simulink model "Cellmodel"  (Simulink 6.6)
settings: Solver=ode4  StartTime=0.0  StopTime=0.0001  FixedStep=0.000000001  RelTol=1e-3
(part 1 of 2)
settings Model: Creator=Thang M. Hoang  LastModifiedBy=Thang M. Hoang

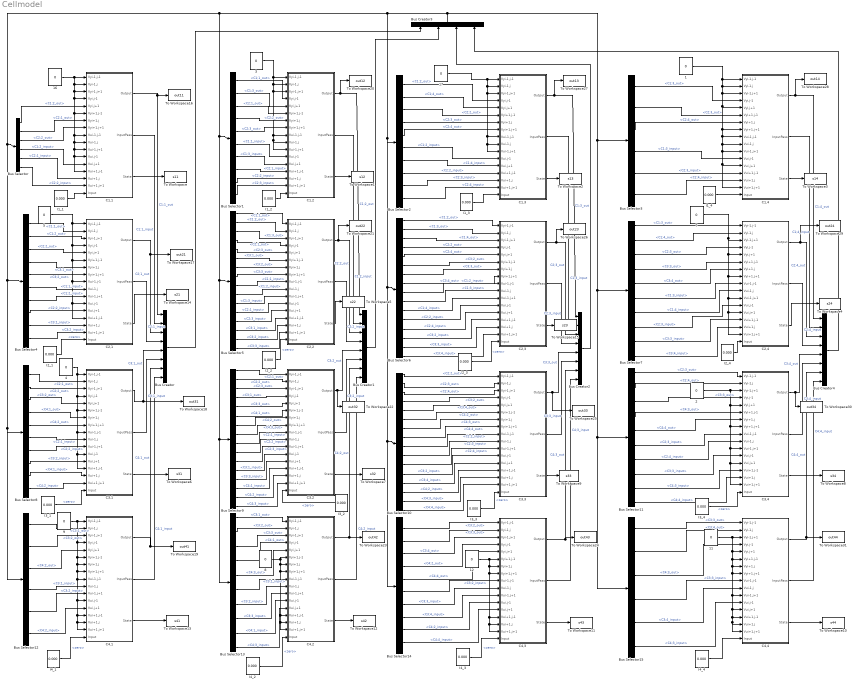
== system Cellmodel ==
  {1..5,7..9,11..12,16..17} (12 alike) : Constant  Value=0
  Bus Creator{,1..2,4} (4 alike) : BusCreator  Inputs=8
  Bus Creator3 : BusCreator  Orientation=up
  Bus Selector : BusSelector  OutputSignals=signal2.C1;2_out,signal1.C2;1_out,signal2.C2;2_out,signal2.C1;2_input,signal1.C2;1_input,signal2.C2;2_input
  Bus Selector1 : BusSelector  OutputSignals=signal1.C1;1_out,signal3.C1;3_out,signal1.C2;1_out,signal2.C2;2_out,signal3.C2;3_out,signal1.C1;1_input,signal3.C1;3_input,signal1.C2;1_input,signal2.C2;2_input,signal3.C2;3_input
  Bus Selector10 : BusSelector  OutputSignals=signal2.C2;2_out,signal3.C2;3_out,signal4.C2;4_out,signal2.C3;2_out,signal4.C3;4_out,signal2.C4;2_out,signal3.C4;3_out,signal4.C4;4_out,signal2.C2;2_input,signal3.C2;3_input,signal4.C2;4_input,signal2.C3;2_input,signal4.C3;4_input,signal2.C4;2_input,signal3.C4;3_input,signal4.C4;4_input
  Bus Selector11 : BusSelector  OutputSignals=signal3.C2;3_out,signal4.C2;4_out,signal3.C3;3_out,signal3.C4;3_out,signal4.C4;4_out,signal3.C2;3_input,signal4.C2;4_input,signal3.C3;3_input,signal3.C4;3_input,signal4.C4;4_input
  Bus Selector12 : BusSelector  OutputSignals=signal1.C3;1_out,signal2.C3;2_out,signal2.C4;2_out,signal1.C3;1_input,signal2.C3;2_input,signal2.C4;2_input
  Bus Selector13 : BusSelector  OutputSignals=signal1.C3;1_out,signal2.C3;2_out,signal3.C3;3_out,signal1.C4;1_out,signal3.C4;3_out,signal1.C3;1_input,signal2.C3;2_input,signal3.C3;3_input,signal1.C4;1_input,signal3.C4;3_input
  Bus Selector14 : BusSelector  OutputSignals=signal2.C3;2_out,signal3.C3;3_out,signal4.C3;4_out,signal2.C4;2_out,signal4.C4;4_out,signal2.C3;2_input,signal3.C3;3_input,signal4.C3;4_input,signal2.C4;2_input,signal4.C4;4_input
  Bus Selector15 : BusSelector  OutputSignals=signal3.C3;3_out,signal4.C3;4_out,signal3.C4;3_out,signal3.C3;3_input,signal4.C3;4_input,signal3.C4;3_input
  Bus Selector2 : BusSelector  OutputSignals=signal2.C1;2_out,signal4.C1;4_out,signal2.C2;2_out,signal3.C2;3_out,signal4.C2;4_out,signal2.C1;2_input,signal4.C1;4_input,signal2.C2;2_input,signal3.C2;3_input,signal4.C2;4_input
  Bus Selector3 : BusSelector  OutputSignals=signal3.C1;3_out,signal3.C2;3_out,signal4.C2;4_out,signal3.C1;3_input,signal3.C2;3_input,signal4.C2;4_input
  Bus Selector4 : BusSelector  OutputSignals=signal1.C1;1_out,signal2.C1;2_out,signal2.C2;2_out,signal1.C3;1_out,signal2.C3;2_out,signal1.C1;1_input,signal2.C1;2_input,signal2.C2;2_input,signal1.C3;1_input,signal2.C3;2_input
  Bus Selector5 : BusSelector  OutputSignals=signal1.C1;1_out,signal2.C1;2_out,signal3.C1;3_out,signal1.C2;1_out,signal3.C2;3_out,signal1.C3;1_out,signal2.C3;2_out,signal3.C3;3_out,signal1.C1;1_input,signal2.C1;2_input,signal3.C1;3_input,signal1.C2;1_input,signal3.C2;3_input,signal1.C3;1_input,signal2.C3;2_input,signal3.C3;3_input
  Bus Selector6 : BusSelector  OutputSignals=signal2.C1;2_out,signal3.C1;3_out,signal4.C1;4_out,signal2.C2;2_out,signal4.C2;4_out,signal2.C3;2_out,signal3.C3;3_out,signal4.C3;4_out,signal2.C1;2_input,signal3.C1;3_input,signal4.C1;4_input,signal2.C2;2_input,signal4.C2;4_input,signal2.C3;2_input,signal3.C3;3_input,signal4.C3;4_input
  Bus Selector7 : BusSelector  OutputSignals=signal3.C1;3_out,signal4.C1;4_out,signal3.C2;3_out,signal3.C3;3_out,signal4.C3;4_out,signal3.C1;3_input,signal4.C1;4_input,signal3.C2;3_input,signal3.C3;3_input,signal4.C3;4_input
  Bus Selector8 : BusSelector  OutputSignals=signal1.C2;1_out,signal2.C2;2_out,signal2.C3;2_out,signal1.C4;1_out,signal2.C4;2_out,signal1.C2;1_input,signal2.C2;2_input,signal2.C3;2_input,signal1.C4;1_input,signal2.C4;2_input
  Bus Selector9 : BusSelector  OutputSignals=signal1.C2;1_out,signal2.C2;2_out,signal3.C2;3_out,signal1.C3;1_out,signal3.C3;3_out,signal1.C4;1_out,signal2.C4;2_out,signal3.C4;3_out,signal1.C2;1_input,signal2.C2;2_input,signal3.C2;3_input,signal1.C3;1_input,signal3.C3;3_input,signal1.C4;1_input,signal2.C4;2_input,signal3.C4;3_input
  C1,1 : Subsystem
  C1,2 : Subsystem
  C1,3 : Subsystem
  C1,4 : Subsystem
  C2,1 : Subsystem
  C2,2 : Subsystem
  C2,3 : Subsystem
  C2,4 : Subsystem
  C3,1 : Subsystem
  C3,2 : Subsystem
  C3,3 : Subsystem
  C3,4 : Subsystem
  C4,1 : Subsystem
  C4,2 : Subsystem
  C4,3 : Subsystem
  C4,4 : Subsystem
  I1_{1..4} (4 alike) : Constant  Value=0.000
  I2_{1..4} (4 alike) : Constant  Value=0.000
  I3_1 : Constant  Value=0.000
  I3_2 : Constant  Orientation=left  Value=0.000
  I3_3 : Constant  Value=0.000
  I3_4 : Constant  Value=0.000
  I4_{1..4} (4 alike) : Constant  Value=0.000
  To Workspace : ToWorkspace  VariableName=s11  SampleTime=-1  SaveFormat=Array
  To Workspace1 : ToWorkspace  VariableName=s12  SampleTime=-1  SaveFormat=Array
  To Workspace10 : ToWorkspace  VariableName=s44  SampleTime=-1  SaveFormat=Array
  To Workspace11 : ToWorkspace  VariableName=s43  SampleTime=-1  SaveFormat=Array
  To Workspace12 : ToWorkspace  VariableName=s42  SampleTime=-1  SaveFormat=Array
  To Workspace13 : ToWorkspace  VariableName=s41  SampleTime=-1  SaveFormat=Array
  To Workspace14 : ToWorkspace  VariableName=s21  SampleTime=-1  SaveFormat=Array
  To Workspace15 : ToWorkspace  VariableName=s23  SampleTime=-1  SaveFormat=Array
  To Workspace16 : ToWorkspace  VariableName=out11  SampleTime=-1  SaveFormat=Array
  To Workspace17 : ToWorkspace  VariableName=out21  SampleTime=-1  SaveFormat=Array
  To Workspace18 : ToWorkspace  VariableName=out31  SampleTime=-1  SaveFormat=Array
  To Workspace19 : ToWorkspace  VariableName=out41  SampleTime=-1  SaveFormat=Array
  To Workspace2 : ToWorkspace  VariableName=s13  SampleTime=-1  SaveFormat=Array
  To Workspace20 : ToWorkspace  VariableName=out12  SampleTime=-1  SaveFormat=Array
  To Workspace21 : ToWorkspace  VariableName=out22  SampleTime=-1  SaveFormat=Array
  To Workspace22 : ToWorkspace  VariableName=out32  SampleTime=-1  SaveFormat=Array
  To Workspace23 : ToWorkspace  VariableName=out42  SampleTime=-1  SaveFormat=Array
  To Workspace24 : ToWorkspace  VariableName=out43  SampleTime=-1  SaveFormat=Array
  To Workspace25 : ToWorkspace  VariableName=out33  SampleTime=-1  SaveFormat=Array
  To Workspace26 : ToWorkspace  VariableName=out23  SampleTime=-1  SaveFormat=Array
  To Workspace27 : ToWorkspace  VariableName=out13  SampleTime=-1  SaveFormat=Array
  To Workspace28 : ToWorkspace  VariableName=out14  SampleTime=-1  SaveFormat=Array
  To Workspace29 : ToWorkspace  VariableName=out24  SampleTime=-1  SaveFormat=Array
  To Workspace3 : ToWorkspace  VariableName=s14  SampleTime=-1  SaveFormat=Array
  To Workspace30 : ToWorkspace  VariableName=out34  SampleTime=-1  SaveFormat=Array
  To Workspace31 : ToWorkspace  VariableName=out44  SampleTime=-1  SaveFormat=Array
  To Workspace4 : ToWorkspace  VariableName=s24  SampleTime=-1  SaveFormat=Array
  To Workspace5 : ToWorkspace  VariableName=s22  SampleTime=-1  SaveFormat=Array
  To Workspace6 : ToWorkspace  VariableName=s31  SampleTime=-1  SaveFormat=Array
  To Workspace7 : ToWorkspace  VariableName=s32  SampleTime=-1  SaveFormat=Array
  To Workspace8 : ToWorkspace  VariableName=s34  SampleTime=-1  SaveFormat=Array
  To Workspace9 : ToWorkspace  VariableName=s33  SampleTime=-1  SaveFormat=Array
  wires:
  C1,1/1(Output) -> Bus Creator/1, To Workspace16/1  "C1;1_out"
  C1,1/2(InputPass) -> Bus Creator/2  "C1;1_input"
  C2,1/1(Output) -> Bus Creator/3, To Workspace17/1  "C2;1_out"
  C2,1/2(InputPass) -> Bus Creator/4  "C2;1_input"
  C3,1/1(Output) -> Bus Creator/5, To Workspace18/1  "C3;1_out"
  C3,1/2(InputPass) -> Bus Creator/6  "C3;1_input"
  C4,1/1(Output) -> Bus Creator/7, To Workspace19/1  "C4;1_out"
  C4,1/2(InputPass) -> Bus Creator/8  "C4;1_input"
  C1,2/1(Output) -> Bus Creator1/1, To Workspace20/1  "C1;2_out"
  C1,2/2(InputPass) -> Bus Creator1/2  "C1;2_input"
  C2,2/1(Output) -> Bus Creator1/3, To Workspace21/1  "C2;2_out"
  C2,2/2(InputPass) -> Bus Creator1/4  "C2;2_input"
  C3,2/1(Output) -> Bus Creator1/5, To Workspace22/1  "C3;2_out"
  C3,2/2(InputPass) -> Bus Creator1/6  "C3;2_input"
  C4,2/1(Output) -> Bus Creator1/7, To Workspace23/1  "C4;2_out"
  C4,2/2(InputPass) -> Bus Creator1/8  "C4;2_input"
  C1,3/1(Output) -> Bus Creator2/1, To Workspace27/1  "C1;3_out"
  C1,3/2(InputPass) -> Bus Creator2/2  "C1;3_input"
  C2,3/1(Output) -> Bus Creator2/3, To Workspace26/1  "C2;3_out"
  C2,3/2(InputPass) -> Bus Creator2/4  "C2;3_input"
  C3,3/1(Output) -> Bus Creator2/5, To Workspace25/1  "C3;3_out"
  C3,3/2(InputPass) -> Bus Creator2/6  "C3;3_input"
  C4,3/1(Output) -> Bus Creator2/7, To Workspace24/1  "C4;3_out"
  C4,3/2(InputPass) -> Bus Creator2/8  "C4;3_input"
  C1,4/1(Output) -> Bus Creator4/1, To Workspace28/1  "C1;4_out"
  C1,4/2(InputPass) -> Bus Creator4/2  "C1;4_input"
  C2,4/1(Output) -> Bus Creator4/3, To Workspace29/1  "C2;4_out"
  C2,4/2(InputPass) -> Bus Creator4/4  "C2;4_input"
  C3,4/1(Output) -> Bus Creator4/5, To Workspace30/1  "C3;4_out"
  C3,4/2(InputPass) -> Bus Creator4/6  "C3;4_input"
  C4,4/1(Output) -> Bus Creator4/7, To Workspace31/1  "C4;4_out"
  C4,4/2(InputPass) -> Bus Creator4/8  "C4;4_input"
  Bus Creator/1 -> Bus Creator3/1
  Bus Creator1/1 -> Bus Creator3/2
  Bus Creator2/1 -> Bus Creator3/3
  Bus Creator4/1 -> Bus Creator3/4
  Bus Creator3/1 -> Bus Selector/1, Bus Selector4/1, Bus Selector8/1, Bus Selector12/1, Bus Selector1/1, Bus Selector5/1, Bus Selector9/1, Bus Selector13/1, Bus Selector2/1, Bus Selector6/1, Bus Selector10/1, Bus Selector14/1, Bus Selector3/1, Bus Selector7/1, Bus Selector11/1, Bus Selector15/1
  Bus Selector/2 -> C1,1/7(Vyi+1,j)  "<C2;1_out>"
  Bus Selector/5 -> C1,1/15(Vui+1,j)  "<C2;1_input>"
  Bus Selector/1 -> C1,1/5(Vyi,j+1)  "<C1;2_out>"
  Bus Selector/4 -> C1,1/13(Vui,j+1)  "<C1;2_input>"
  Bus Selector/3 -> C1,1/8(Vyi+1,j+1)  "<C2;2_out>"
  Bus Selector/6 -> C1,1/16(Vui+1,j+1)  "<C2;2_input>"
  Bus Selector1/1 -> C1,2/4(Vyi,j-1)  "<C1;1_out>"
  Bus Selector1/6 -> C1,2/12(Vui,j-1)  "<C1;1_input>"
  Bus Selector1/3 -> C1,2/6(Vyi+1,j-1)  "<C2;1_out>"
  Bus Selector1/8 -> C1,2/14(Vui+1,j-1)  "<C2;1_input>"
  Bus Selector1/4 -> C1,2/7(Vyi+1,j)  "<C2;2_out>"
  Bus Selector1/9 -> C1,2/15(Vui+1,j)  "<C2;2_input>"
  Bus Selector1/2 -> C1,2/5(Vyi,j+1)  "<C1;3_out>"
  Bus Selector1/7 -> C1,2/13(Vui,j+1)  "<C1;3_input>"
  Bus Selector1/5 -> C1,2/8(Vyi+1,j+1)  "<C2;3_out>"
  Bus Selector1/10 -> C1,2/16(Vui+1,j+1)  "<C2;3_input>"
  Bus Selector2/1 -> C1,3/4(Vyi,j-1)  "<C1;2_out>"
  Bus Selector2/3 -> C1,3/6(Vyi+1,j-1)  "<C2;2_out>"
  Bus Selector2/4 -> C1,3/7(Vyi+1,j)  "<C2;3_out>"
  Bus Selector2/2 -> C1,3/5(Vyi,j+1)  "<C1;4_out>"
  Bus Selector2/5 -> C1,3/8(Vyi+1,j+1)  "<C2;4_out>"
  Bus Selector2/6 -> C1,3/12(Vui,j-1)  "<C1;2_input>"
  Bus Selector2/8 -> C1,3/14(Vui+1,j-1)  "<C2;2_input>"
  Bus Selector2/9 -> C1,3/15(Vui+1,j)  "<C2;3_input>"
  Bus Selector2/7 -> C1,3/13(Vui,j+1)  "<C1;4_input>"
  Bus Selector2/10 -> C1,3/16(Vui+1,j+1)  "<C2;4_input>"
  Bus Selector3/1 -> C1,4/4(Vyi,j-1)  "<C1;3_out>"
  Bus Selector3/2 -> C1,4/6(Vyi+1,j-1)  "<C2;3_out>"
  Bus Selector3/3 -> C1,4/7(Vyi+1,j)  "<C2;4_out>"
  Bus Selector3/4 -> C1,4/12(Vui,j-1)  "<C1;3_input>"
  Bus Selector3/5 -> C1,4/14(Vui+1,j-1)  "<C2;3_input>"
  Bus Selector3/6 -> C1,4/15(Vui+1,j)  "<C2;4_input>"
  Bus Selector4/1 -> C2,1/2(Vyi-1,j)  "<C1;1_out>"
  Bus Selector4/4 -> C2,1/7(Vyi+1,j)  "<C3;1_out>"
  Bus Selector4/2 -> C2,1/3(Vyi-1,j+1)  "<C1;2_out>"
  Bus Selector4/3 -> C2,1/5(Vyi,j+1)  "<C2;2_out>"
  Bus Selector4/5 -> C2,1/8(Vyi+1,j+1)  "<C3;2_out>"
  Bus Selector4/6 -> C2,1/10(Vui-1,j)  "<C1;1_input>"
  Bus Selector4/9 -> C2,1/15(Vui+1,j)  "<C3;1_input>"
  Bus Selector4/7 -> C2,1/11(Vui-1,j+1)  "<C1;2_input>"
  Bus Selector4/8 -> C2,1/13(Vui,j+1)  "<C2;2_input>"
  Bus Selector4/10 -> C2,1/16(Vui+1,j+1)  "<C3;2_input>"
  Bus Selector5/1 -> C2,2/1(Vyi-1,j-1)  "<C1;1_out>"
  Bus Selector5/4 -> C2,2/4(Vyi,j-1)  "<C2;1_out>"
  Bus Selector5/6 -> C2,2/6(Vyi+1,j-1)  "<C3;1_out>"
  Bus Selector5/2 -> C2,2/2(Vyi-1,j)  "<C1;2_out>"
  Bus Selector5/7 -> C2,2/7(Vyi+1,j)  "<C3;2_out>"
  Bus Selector5/3 -> C2,2/3(Vyi-1,j+1)  "<C1;3_out>"
  Bus Selector5/5 -> C2,2/5(Vyi,j+1)  "<C2;3_out>"
  Bus Selector5/8 -> C2,2/8(Vyi+1,j+1)  "<C3;3_out>"
  Bus Selector5/9 -> C2,2/9(Vui-1,j-1)  "<C1;1_input>"
  Bus Selector5/10 -> C2,2/10(Vui-1,j)  "<C1;2_input>"
  Bus Selector5/11 -> C2,2/11(Vui-1,j+1)  "<C1;3_input>"
  Bus Selector5/12 -> C2,2/12(Vui,j-1)  "<C2;1_input>"
  Bus Selector5/13 -> C2,2/13(Vui,j+1)  "<C2;3_input>"
  Bus Selector5/14 -> C2,2/14(Vui+1,j-1)  "<C3;1_input>"
  Bus Selector5/15 -> C2,2/15(Vui+1,j)  "<C3;2_input>"
  Bus Selector5/16 -> C2,2/16(Vui+1,j+1)  "<C3;3_input>"
  Bus Selector6/1 -> C2,3/1(Vyi-1,j-1)  "<C1;2_out>"
  Bus Selector6/4 -> C2,3/4(Vyi,j-1)  "<C2;2_out>"
  Bus Selector6/6 -> C2,3/6(Vyi+1,j-1)  "<C3;2_out>"
  Bus Selector6/2 -> C2,3/2(Vyi-1,j)  "<C1;3_out>"
  Bus Selector6/7 -> C2,3/7(Vyi+1,j)  "<C3;3_out>"
  Bus Selector6/3 -> C2,3/3(Vyi-1,j+1)  "<C1;4_out>"
  Bus Selector6/5 -> C2,3/5(Vyi,j+1)  "<C2;4_out>"
  Bus Selector6/8 -> C2,3/8(Vyi+1,j+1)  "<C3;4_out>"
  Bus Selector6/9 -> C2,3/9(Vui-1,j-1)  "<C1;2_input>"
  Bus Selector6/10 -> C2,3/10(Vui-1,j)  "<C1;3_input>"
  Bus Selector6/11 -> C2,3/11(Vui-1,j+1)  "<C1;4_input>"
  Bus Selector6/16 -> C2,3/16(Vui+1,j+1)  "<C3;4_input>"
  Bus Selector6/12 -> C2,3/12(Vui,j-1)  "<C2;2_input>"
  Bus Selector6/13 -> C2,3/13(Vui,j+1)  "<C2;4_input>"
  Bus Selector6/14 -> C2,3/14(Vui+1,j-1)  "<C3;2_input>"
  Bus Selector6/15 -> C2,3/15(Vui+1,j)  "<C3;3_input>"
  Bus Selector7/1 -> C2,4/1(Vyi-1,j-1)  "<C1;3_out>"
  Bus Selector7/2 -> C2,4/2(Vyi-1,j)  "<C1;4_out>"
  Bus Selector7/3 -> C2,4/4(Vyi,j-1)  "<C2;3_out>"
  Bus Selector7/4 -> C2,4/6(Vyi+1,j-1)  "<C3;3_out>"
  Bus Selector7/5 -> C2,4/7(Vyi+1,j)  "<C3;4_out>"
  Bus Selector7/8 -> C2,4/12(Vui,j-1)  "<C2;3_input>"
  Bus Selector7/6 -> C2,4/9(Vui-1,j-1)  "<C1;3_input>"
  Bus Selector7/7 -> C2,4/10(Vui-1,j)  "<C1;4_input>"
  Bus Selector7/9 -> C2,4/14(Vui+1,j-1)  "<C3;3_input>"
  Bus Selector7/10 -> C2,4/15(Vui+1,j)  "<C3;4_input>"
  Bus Selector8/1 -> C3,1/2(Vyi-1,j)  "<C2;1_out>"
  Bus Selector8/2 -> C3,1/3(Vyi-1,j+1)  "<C2;2_out>"
  Bus Selector8/3 -> C3,1/5(Vyi,j+1)  "<C3;2_out>"
  Bus Selector8/4 -> C3,1/7(Vyi+1,j)  "<C4;1_out>"
  Bus Selector8/5 -> C3,1/8(Vyi+1,j+1)  "<C4;2_out>"
  Bus Selector8/6 -> C3,1/10(Vui-1,j)  "<C2;1_input>"
  Bus Selector8/7 -> C3,1/11(Vui-1,j+1)  "<C2;2_input>"
  Bus Selector8/8 -> C3,1/13(Vui,j+1)  "<C3;2_input>"
  Bus Selector8/9 -> C3,1/15(Vui+1,j)  "<C4;1_input>"
  Bus Selector8/10 -> C3,1/16(Vui+1,j+1)  "<C4;2_input>"
  Bus Selector9/1 -> C3,2/1(Vyi-1,j-1)  "<C2;1_out>"
  Bus Selector9/2 -> C3,2/2(Vyi-1,j)  "<C2;2_out>"
  Bus Selector9/3 -> C3,2/3(Vyi-1,j+1)  "<C2;3_out>"
  Bus Selector9/4 -> C3,2/4(Vyi,j-1)  "<C3;1_out>"
  Bus Selector9/5 -> C3,2/5(Vyi,j+1)  "<C3;3_out>"
  Bus Selector9/6 -> C3,2/6(Vyi+1,j-1)  "<C4;1_out>"
  Bus Selector9/7 -> C3,2/7(Vyi+1,j)  "<C4;2_out>"
  Bus Selector9/8 -> C3,2/8(Vyi+1,j+1)  "<C4;3_out>"
  Bus Selector9/9 -> C3,2/9(Vui-1,j-1)  "<C2;1_input>"
  Bus Selector9/10 -> C3,2/10(Vui-1,j)  "<C2;2_input>"
  Bus Selector9/11 -> C3,2/11(Vui-1,j+1)  "<C2;3_input>"
  Bus Selector9/12 -> C3,2/12(Vui,j-1)  "<C3;1_input>"
  Bus Selector9/13 -> C3,2/13(Vui,j+1)  "<C3;3_input>"
  Bus Selector9/14 -> C3,2/14(Vui+1,j-1)  "<C4;1_input>"
  Bus Selector9/15 -> C3,2/15(Vui+1,j)  "<C4;2_input>"
  Bus Selector9/16 -> C3,2/16(Vui+1,j+1)  "<C4;3_input>"
  Bus Selector10/1 -> C3,3/1(Vyi-1,j-1)  "<C2;2_out>"
  Bus Selector10/2 -> C3,3/2(Vyi-1,j)  "<C2;3_out>"
  Bus Selector10/3 -> C3,3/3(Vyi-1,j+1)  "<C2;4_out>"
  Bus Selector10/4 -> C3,3/4(Vyi,j-1)  "<C3;2_out>"
  Bus Selector10/5 -> C3,3/5(Vyi,j+1)  "<C3;4_out>"
  Bus Selector10/6 -> C3,3/6(Vyi+1,j-1)  "<C4;2_out>"
  Bus Selector10/7 -> C3,3/7(Vyi+1,j)  "<C4;3_out>"
  Bus Selector10/8 -> C3,3/8(Vyi+1,j+1)  "<C4;4_out>"
  Bus Selector10/9 -> C3,3/9(Vui-1,j-1)  "<C2;2_input>"
  Bus Selector10/10 -> C3,3/10(Vui-1,j)  "<C2;3_input>"
  Bus Selector10/11 -> C3,3/11(Vui-1,j+1)  "<C2;4_input>"
  Bus Selector10/12 -> C3,3/12(Vui,j-1)  "<C3;2_input>"
  Bus Selector10/13 -> C3,3/13(Vui,j+1)  "<C3;4_input>"
  Bus Selector10/14 -> C3,3/14(Vui+1,j-1)  "<C4;2_input>"
  Bus Selector10/15 -> C3,3/15(Vui+1,j)  "<C4;3_input>"
  Bus Selector10/16 -> C3,3/16(Vui+1,j+1)  "<C4;4_input>"
  Bus Selector11/1 -> C3,4/1(Vyi-1,j-1)  "<C2;3_out>"
  Bus Selector11/2 -> C3,4/2(Vyi-1,j)  "<C2;4_out>"
  Bus Selector11/3 -> C3,4/4(Vyi,j-1)  "<C3;3_out>"
  Bus Selector11/4 -> C3,4/6(Vyi+1,j-1)  "<C4;3_out>"
  Bus Selector11/5 -> C3,4/7(Vyi+1,j)  "<C4;4_out>"
  Bus Selector11/6 -> C3,4/9(Vui-1,j-1)  "<C2;3_input>"
  Bus Selector11/7 -> C3,4/10(Vui-1,j)  "<C2;4_input>"
  Bus Selector11/8 -> C3,4/12(Vui,j-1)  "<C3;3_input>"
  Bus Selector11/9 -> C3,4/14(Vui+1,j-1)  "<C4;3_input>"
  Bus Selector11/10 -> C3,4/15(Vui+1,j)  "<C4;4_input>"
  Bus Selector12/1 -> C4,1/2(Vyi-1,j)  "<C3;1_out>"
  Bus Selector12/2 -> C4,1/3(Vyi-1,j+1)  "<C3;2_out>"
  Bus Selector12/3 -> C4,1/5(Vyi,j+1)  "<C4;2_out>"
  Bus Selector12/4 -> C4,1/10(Vui-1,j)  "<C3;1_input>"
  Bus Selector12/5 -> C4,1/11(Vui-1,j+1)  "<C3;2_input>"
  Bus Selector12/6 -> C4,1/13(Vui,j+1)  "<C4;2_input>"
  Bus Selector13/1 -> C4,2/1(Vyi-1,j-1)  "<C3;1_out>"
  Bus Selector13/2 -> C4,2/2(Vyi-1,j)  "<C3;2_out>"
  Bus Selector13/3 -> C4,2/3(Vyi-1,j+1)  "<C3;3_out>"
  Bus Selector13/4 -> C4,2/4(Vyi,j-1)  "<C4;1_out>"
  Bus Selector13/5 -> C4,2/5(Vyi,j+1)  "<C4;3_out>"
  Bus Selector13/6 -> C4,2/9(Vui-1,j-1)  "<C3;1_input>"
  Bus Selector13/7 -> C4,2/10(Vui-1,j)  "<C3;2_input>"
  Bus Selector13/8 -> C4,2/11(Vui-1,j+1)  "<C3;3_input>"
  Bus Selector13/9 -> C4,2/12(Vui,j-1)  "<C4;1_input>"
  Bus Selector13/10 -> C4,2/13(Vui,j+1)  "<C4;3_input>"
  Bus Selector14/1 -> C4,3/1(Vyi-1,j-1)  "<C3;2_out>"
  Bus Selector14/2 -> C4,3/2(Vyi-1,j)  "<C3;3_out>"
  Bus Selector14/3 -> C4,3/3(Vyi-1,j+1)  "<C3;4_out>"
  Bus Selector14/4 -> C4,3/4(Vyi,j-1)  "<C4;2_out>"
  Bus Selector14/5 -> C4,3/5(Vyi,j+1)  "<C4;4_out>"
  Bus Selector14/6 -> C4,3/9(Vui-1,j-1)  "<C3;2_input>"
  Bus Selector14/7 -> C4,3/10(Vui-1,j)  "<C3;3_input>"
  Bus Selector14/8 -> C4,3/11(Vui-1,j+1)  "<C3;4_input>"
  Bus Selector14/9 -> C4,3/12(Vui,j-1)  "<C4;2_input>"
  Bus Selector14/10 -> C4,3/13(Vui,j+1)  "<C4;4_input>"
  Bus Selector15/1 -> C4,4/1(Vyi-1,j-1)  "<C3;3_out>"
  Bus Selector15/2 -> C4,4/2(Vyi-1,j)  "<C3;4_out>"
  Bus Selector15/3 -> C4,4/4(Vyi,j-1)  "<C4;3_out>"
  Bus Selector15/4 -> C4,4/9(Vui-1,j-1)  "<C3;3_input>"
  Bus Selector15/5 -> C4,4/10(Vui-1,j)  "<C3;4_input>"
  Bus Selector15/6 -> C4,4/12(Vui,j-1)  "<C4;3_input>"
  I2_3/1 -> C2,3/17(Input)  "<zero>"
  I2_2/1 -> C2,2/17(Input)  "<zero>"
  I2_1/1 -> C2,1/17(Input)  "<zero>"
  I3_2/1 -> C3,2/17(Input)  "<zero>"
  I3_3/1 -> C3,3/17(Input)  "<zero>"
  16/1 -> C1,1/1(Vyi-1,j-1), C1,1/2(Vyi-1,j), C1,1/3(Vyi-1,j+1), C1,1/4(Vyi,j-1), C1,1/6(Vyi+1,j-1), C1,1/9(Vui-1,j-1), C1,1/10(Vui-1,j), C1,1/11(Vui-1,j+1), C1,1/12(Vui,j-1), C1,1/14(Vui+1,j-1)
  I1_1/1 -> C1,1/17(Input)
  I1_2/1 -> C1,2/17(Input)
  3/1 -> C1,2/1(Vyi-1,j-1), C1,2/2(Vyi-1,j), C1,2/3(Vyi-1,j+1), C1,2/9(Vui-1,j-1), C1,2/10(Vui-1,j), C1,2/11(Vui-1,j+1)
  I1_3/1 -> C1,3/17(Input)
  17/1 -> C1,3/1(Vyi-1,j-1), C1,3/2(Vyi-1,j), C1,3/3(Vyi-1,j+1), C1,3/9(Vui-1,j-1), C1,3/10(Vui-1,j), C1,3/11(Vui-1,j+1)
  I1_4/1 -> C1,4/17(Input)
  1/1 -> C1,4/1(Vyi-1,j-1), C1,4/2(Vyi-1,j), C1,4/3(Vyi-1,j+1), C1,4/5(Vyi,j+1), C1,4/8(Vyi+1,j+1), C1,4/9(Vui-1,j-1), C1,4/10(Vui-1,j), C1,4/11(Vui-1,j+1), C1,4/13(Vui,j+1), C1,4/16(Vui+1,j+1)
  7/1 -> C2,4/3(Vyi-1,j+1), C2,4/11(Vui-1,j+1), C2,4/13(Vui,j+1), C2,4/16(Vui+1,j+1), C2,4/8(Vyi+1,j+1), C2,4/5(Vyi,j+1)
  I2_4/1 -> C2,4/17(Input)
  2/1 -> C3,4/3(Vyi-1,j+1), C3,4/5(Vyi,j+1), C3,4/8(Vyi+1,j+1), C3,4/11(Vui-1,j+1), C3,4/13(Vui,j+1), C3,4/16(Vui+1,j+1)
  I3_4/1 -> C3,4/17(Input)  "<zero>"
  11/1 -> C4,4/3(Vyi-1,j+1), C4,4/5(Vyi,j+1), C4,4/6(Vyi+1,j-1), C4,4/7(Vyi+1,j), C4,4/8(Vyi+1,j+1), C4,4/11(Vui-1,j+1), C4,4/13(Vui,j+1), C4,4/14(Vui+1,j-1), C4,4/15(Vui+1,j), C4,4/16(Vui+1,j+1)
  I4_4/1 -> C4,4/17(Input)
  12/1 -> C4,3/6(Vyi+1,j-1), C4,3/7(Vyi+1,j), C4,3/8(Vyi+1,j+1), C4,3/14(Vui+1,j-1), C4,3/15(Vui+1,j), C4,3/16(Vui+1,j+1)
  I4_3/1 -> C4,3/17(Input)  "<zero>"
  5/1 -> C2,1/1(Vyi-1,j-1), C2,1/4(Vyi,j-1), C2,1/6(Vyi+1,j-1), C2,1/9(Vui-1,j-1), C2,1/12(Vui,j-1), C2,1/14(Vui+1,j-1)
  4/1 -> C3,1/1(Vyi-1,j-1), C3,1/4(Vyi,j-1), C3,1/6(Vyi+1,j-1), C3,1/9(Vui-1,j-1), C3,1/12(Vui,j-1), C3,1/14(Vui+1,j-1)
  I3_1/1 -> C3,1/17(Input)  "<zero>"
  8/1 -> C4,2/6(Vyi+1,j-1), C4,2/7(Vyi+1,j), C4,2/8(Vyi+1,j+1), C4,2/14(Vui+1,j-1), C4,2/15(Vui+1,j), C4,2/16(Vui+1,j+1)
  I4_2/1 -> C4,2/17(Input)  "<zero>"
  9/1 -> C4,1/1(Vyi-1,j-1), C4,1/4(Vyi,j-1), C4,1/6(Vyi+1,j-1), C4,1/7(Vyi+1,j), C4,1/8(Vyi+1,j+1), C4,1/9(Vui-1,j-1), C4,1/12(Vui,j-1), C4,1/14(Vui+1,j-1), C4,1/15(Vui+1,j), C4,1/16(Vui+1,j+1)
  I4_1/1 -> C4,1/17(Input)  "<zero>"
  C1,1/3(State) -> To Workspace/1
  C2,1/3(State) -> To Workspace14/1
  C3,1/3(State) -> To Workspace6/1
  C4,1/3(State) -> To Workspace13/1
  C4,2/3(State) -> To Workspace12/1
  C3,2/3(State) -> To Workspace7/1
  C2,2/3(State) -> To Workspace5/1
  C1,2/3(State) -> To Workspace1/1
  C1,3/3(State) -> To Workspace2/1
  C2,3/3(State) -> To Workspace15/1
  C3,3/3(State) -> To Workspace9/1
  C4,3/3(State) -> To Workspace11/1
  C4,4/3(State) -> To Workspace10/1
  C3,4/3(State) -> To Workspace8/1
  C2,4/3(State) -> To Workspace4/1
  C1,4/3(State) -> To Workspace3/1

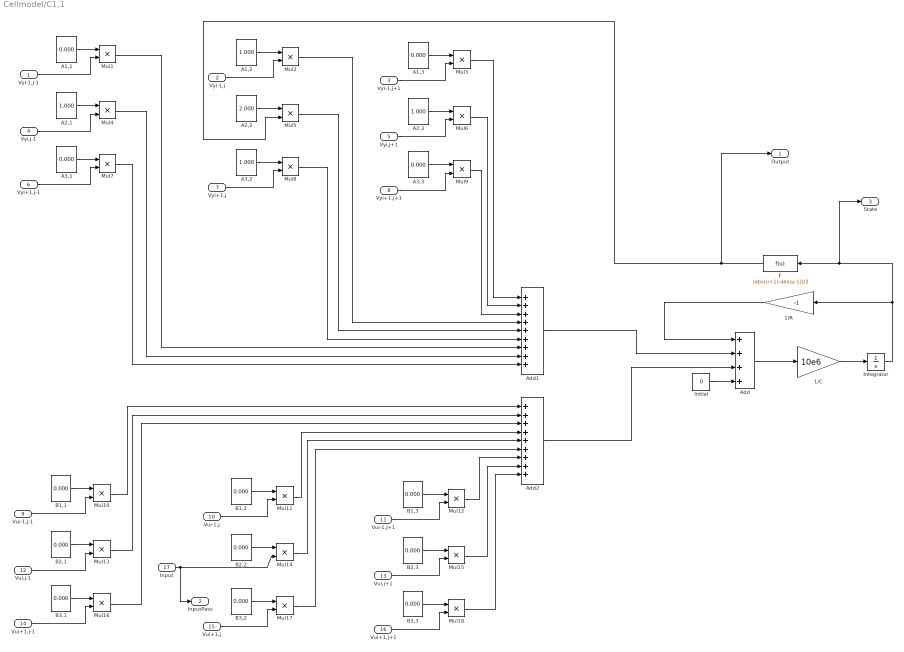
== system Cellmodel/C1,1 ==
  Vyi-1,j-1 : Inport
  Vyi-1,j : Inport  Port=2
  Vyi-1,j+1 : Inport  Port=3
  Vyi,j-1 : Inport  Port=4
  Vyi,j+1 : Inport  Port=5
  Vyi+1,j-1 : Inport  Port=6
  Vyi+1,j : Inport  Port=7
  Vyi+1,j+1 : Inport  Port=8
  Vui-1,j-1 : Inport  Port=9
  Vui-1,j : Inport  Port=10
  Vui-1,j+1 : Inport  Port=11
  Vui,j-1 : Inport  Port=12
  Vui,j+1 : Inport  Port=13
  Vui+1,j-1 : Inport  Port=14
  Vui+1,j : Inport  Port=15
  Vui+1,j+1 : Inport  Port=16
  Input : Inport  Port=17
  1/C : Gain  Gain=10e6
  1/R : Gain  Orientation=left  Gain=-1
  A1,1 : Constant  Value=0.000
  A1,2 : Constant  Value=1.000
  A1,3 : Constant  Value=0.000
  A2,1 : Constant  Value=1.000
  A2,2 : Constant  Value=2.000
  A2,3 : Constant  Value=1.000
  A3,1 : Constant  Value=0.000
  A3,2 : Constant  Value=1.000
  A3,3 : Constant  Value=0.000
  Add : Sum  Inputs=++++  OutScaling=2^-10
  Add1 : Sum  Inputs=+++++++++  OutScaling=2^-10
  Add2 : Sum  Inputs=+++++++++  OutScaling=2^-10
  B1,1 : Constant  Value=0.000
  B1,2 : Constant  Value=0.000
  B1,3 : Constant  Value=0.000
  B2,1 : Constant  Value=0.000
  B2,2 : Constant  Value=0.000
  B2,3 : Constant  Value=0.000
  B3,1 : Constant  Value=0.000
  B3,2 : Constant  Value=0.000
  B3,3 : Constant  Value=0.000
  F : Fcn  Orientation=left  Expr=(abs(u+1)-abs(u-1))/2
  Initial : Constant  Value=0
  Integrator : Integrator  InitialCondition=-0.800
  Mul{1..18} (18 alike) : Product  Inputs=**  OutScaling=2^-10
  Output : Outport
  InputPass : Outport  Port=2
  State : Outport  Port=3
  wires:
  Add/1 -> 1/C/1
  1/C/1 -> Integrator/1
  Initial/1 -> Add/4
  1/R/1 -> Add/1
  Integrator/1 -> 1/R/1, F/1, State/1
  A1,1/1 -> Mul1/1
  Vyi-1,j-1/1 -> Mul1/2
  A1,2/1 -> Mul2/1
  Vyi-1,j/1 -> Mul2/2
  A1,3/1 -> Mul3/1
  Vyi-1,j+1/1 -> Mul3/2
  A2,1/1 -> Mul4/1
  Vyi,j-1/1 -> Mul4/2
  A2,2/1 -> Mul5/1
  A2,3/1 -> Mul6/1
  Vyi,j+1/1 -> Mul6/2
  A3,1/1 -> Mul7/1
  Vyi+1,j-1/1 -> Mul7/2
  A3,2/1 -> Mul8/1
  Vyi+1,j/1 -> Mul8/2
  A3,3/1 -> Mul9/1
  Vyi+1,j+1/1 -> Mul9/2
  F/1 -> Mul5/2, Output/1
  Mul3/1 -> Add1/1
  Mul6/1 -> Add1/2
  Mul9/1 -> Add1/3
  Mul2/1 -> Add1/4
  Mul5/1 -> Add1/5
  Mul8/1 -> Add1/6
  Mul1/1 -> Add1/7
  Mul4/1 -> Add1/8
  Mul7/1 -> Add1/9
  Add1/1 -> Add/2
  B1,1/1 -> Mul10/1
  Vui-1,j-1/1 -> Mul10/2
  B1,2/1 -> Mul11/1
  Vui-1,j/1 -> Mul11/2
  B1,3/1 -> Mul12/1
  Vui-1,j+1/1 -> Mul12/2
  B2,1/1 -> Mul13/1
  Vui,j-1/1 -> Mul13/2
  B2,2/1 -> Mul14/1
  B2,3/1 -> Mul15/1
  Vui,j+1/1 -> Mul15/2
  B3,1/1 -> Mul16/1
  Vui+1,j-1/1 -> Mul16/2
  B3,2/1 -> Mul17/1
  Vui+1,j/1 -> Mul17/2
  B3,3/1 -> Mul18/1
  Vui+1,j+1/1 -> Mul18/2
  Mul10/1 -> Add2/1
  Mul13/1 -> Add2/2
  Mul16/1 -> Add2/3
  Mul11/1 -> Add2/4
  Mul14/1 -> Add2/5
  Mul17/1 -> Add2/6
  Mul12/1 -> Add2/7
  Mul15/1 -> Add2/8
  Mul18/1 -> Add2/9
  Input/1 -> Mul14/2, InputPass/1
  Add2/1 -> Add/3

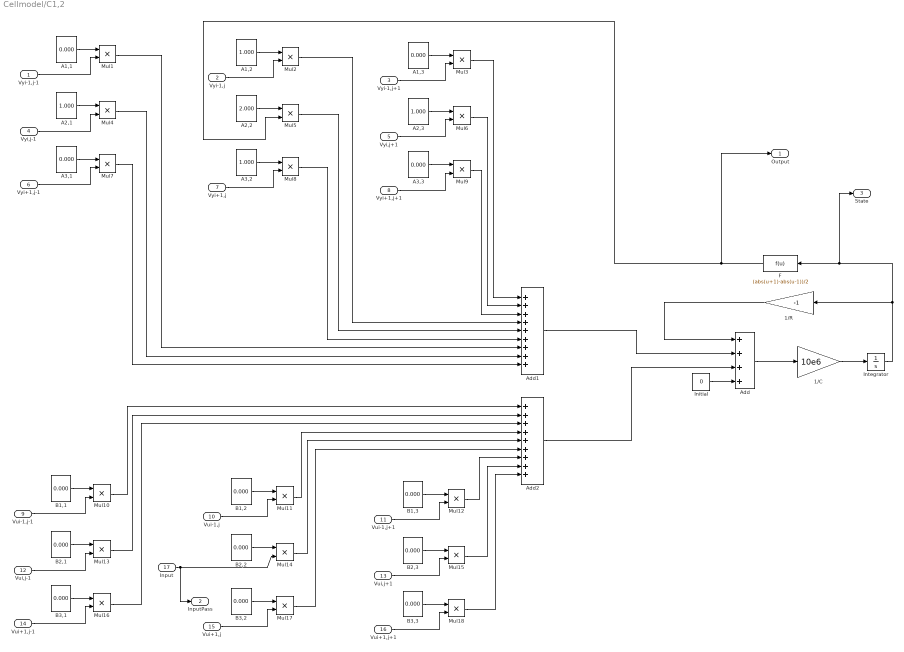
== system Cellmodel/C1,2 ==
  Vyi-1,j-1 : Inport
  Vyi-1,j : Inport  Port=2
  Vyi-1,j+1 : Inport  Port=3
  Vyi,j-1 : Inport  Port=4
  Vyi,j+1 : Inport  Port=5
  Vyi+1,j-1 : Inport  Port=6
  Vyi+1,j : Inport  Port=7
  Vyi+1,j+1 : Inport  Port=8
  Vui-1,j-1 : Inport  Port=9
  Vui-1,j : Inport  Port=10
  Vui-1,j+1 : Inport  Port=11
  Vui,j-1 : Inport  Port=12
  Vui,j+1 : Inport  Port=13
  Vui+1,j-1 : Inport  Port=14
  Vui+1,j : Inport  Port=15
  Vui+1,j+1 : Inport  Port=16
  Input : Inport  Port=17
  1/C : Gain  Gain=10e6
  1/R : Gain  Orientation=left  Gain=-1
  A1,1 : Constant  Value=0.000
  A1,2 : Constant  Value=1.000
  A1,3 : Constant  Value=0.000
  A2,1 : Constant  Value=1.000
  A2,2 : Constant  Value=2.000
  A2,3 : Constant  Value=1.000
  A3,1 : Constant  Value=0.000
  A3,2 : Constant  Value=1.000
  A3,3 : Constant  Value=0.000
  Add : Sum  Inputs=++++  OutScaling=2^-10
  Add1 : Sum  Inputs=+++++++++  OutScaling=2^-10
  Add2 : Sum  Inputs=+++++++++  OutScaling=2^-10
  B1,1 : Constant  Value=0.000
  B1,2 : Constant  Value=0.000
  B1,3 : Constant  Value=0.000
  B2,1 : Constant  Value=0.000
  B2,2 : Constant  Value=0.000
  B2,3 : Constant  Value=0.000
  B3,1 : Constant  Value=0.000
  B3,2 : Constant  Value=0.000
  B3,3 : Constant  Value=0.000
  F : Fcn  Orientation=left  Expr=(abs(u+1)-abs(u-1))/2
  Initial : Constant  Value=0
  Integrator : Integrator  InitialCondition=1.000
  Mul{1..18} (18 alike) : Product  Inputs=**  OutScaling=2^-10
  Output : Outport
  InputPass : Outport  Port=2
  State : Outport  Port=3
  wires:
  Add2/1 -> Add/3
  Input/1 -> InputPass/1, Mul14/2
  Mul18/1 -> Add2/9
  Mul15/1 -> Add2/8
  Mul12/1 -> Add2/7
  Mul17/1 -> Add2/6
  Mul14/1 -> Add2/5
  Mul11/1 -> Add2/4
  Mul16/1 -> Add2/3
  Mul13/1 -> Add2/2
  Mul10/1 -> Add2/1
  Vui+1,j+1/1 -> Mul18/2
  B3,3/1 -> Mul18/1
  Vui+1,j/1 -> Mul17/2
  B3,2/1 -> Mul17/1
  Vui+1,j-1/1 -> Mul16/2
  B3,1/1 -> Mul16/1
  Vui,j+1/1 -> Mul15/2
  B2,3/1 -> Mul15/1
  B2,2/1 -> Mul14/1
  Vui,j-1/1 -> Mul13/2
  B2,1/1 -> Mul13/1
  Vui-1,j+1/1 -> Mul12/2
  B1,3/1 -> Mul12/1
  Vui-1,j/1 -> Mul11/2
  B1,2/1 -> Mul11/1
  Vui-1,j-1/1 -> Mul10/2
  B1,1/1 -> Mul10/1
  Add1/1 -> Add/2
  Mul7/1 -> Add1/9
  Mul4/1 -> Add1/8
  Mul1/1 -> Add1/7
  Mul8/1 -> Add1/6
  Mul5/1 -> Add1/5
  Mul2/1 -> Add1/4
  Mul9/1 -> Add1/3
  Mul6/1 -> Add1/2
  Mul3/1 -> Add1/1
  F/1 -> Mul5/2, Output/1
  Vyi+1,j+1/1 -> Mul9/2
  A3,3/1 -> Mul9/1
  Vyi+1,j/1 -> Mul8/2
  A3,2/1 -> Mul8/1
  Vyi+1,j-1/1 -> Mul7/2
  A3,1/1 -> Mul7/1
  Vyi,j+1/1 -> Mul6/2
  A2,3/1 -> Mul6/1
  A2,2/1 -> Mul5/1
  Vyi,j-1/1 -> Mul4/2
  A2,1/1 -> Mul4/1
  Vyi-1,j+1/1 -> Mul3/2
  A1,3/1 -> Mul3/1
  Vyi-1,j/1 -> Mul2/2
  A1,2/1 -> Mul2/1
  Vyi-1,j-1/1 -> Mul1/2
  A1,1/1 -> Mul1/1
  Integrator/1 -> 1/R/1, F/1, State/1
  1/R/1 -> Add/1
  Initial/1 -> Add/4
  1/C/1 -> Integrator/1
  Add/1 -> 1/C/1

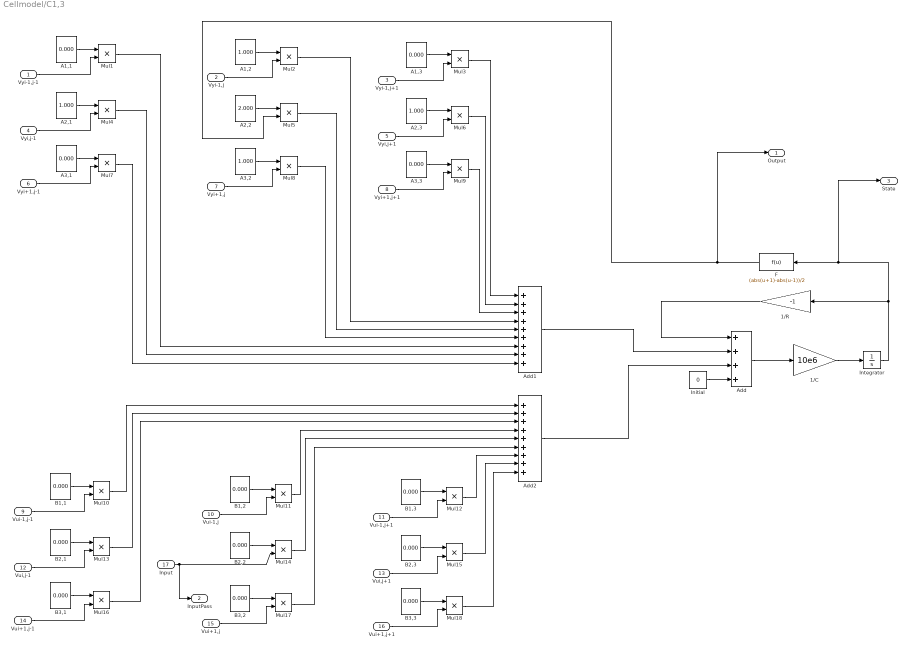
== system Cellmodel/C1,3 ==
  Vyi-1,j-1 : Inport
  Vyi-1,j : Inport  Port=2
  Vyi-1,j+1 : Inport  Port=3
  Vyi,j-1 : Inport  Port=4
  Vyi,j+1 : Inport  Port=5
  Vyi+1,j-1 : Inport  Port=6
  Vyi+1,j : Inport  Port=7
  Vyi+1,j+1 : Inport  Port=8
  Vui-1,j-1 : Inport  Port=9
  Vui-1,j : Inport  Port=10
  Vui-1,j+1 : Inport  Port=11
  Vui,j-1 : Inport  Port=12
  Vui,j+1 : Inport  Port=13
  Vui+1,j-1 : Inport  Port=14
  Vui+1,j : Inport  Port=15
  Vui+1,j+1 : Inport  Port=16
  Input : Inport  Port=17
  1/C : Gain  Gain=10e6
  1/R : Gain  Orientation=left  Gain=-1
  A1,1 : Constant  Value=0.000
  A1,2 : Constant  Value=1.000
  A1,3 : Constant  Value=0.000
  A2,1 : Constant  Value=1.000
  A2,2 : Constant  Value=2.000
  A2,3 : Constant  Value=1.000
  A3,1 : Constant  Value=0.000
  A3,2 : Constant  Value=1.000
  A3,3 : Constant  Value=0.000
  Add : Sum  Inputs=++++  OutScaling=2^-10
  Add1 : Sum  Inputs=+++++++++  OutScaling=2^-10
  Add2 : Sum  Inputs=+++++++++  OutScaling=2^-10
  B1,1 : Constant  Value=0.000
  B1,2 : Constant  Value=0.000
  B1,3 : Constant  Value=0.000
  B2,1 : Constant  Value=0.000
  B2,2 : Constant  Value=0.000
  B2,3 : Constant  Value=0.000
  B3,1 : Constant  Value=0.000
  B3,2 : Constant  Value=0.000
  B3,3 : Constant  Value=0.000
  F : Fcn  Orientation=left  Expr=(abs(u+1)-abs(u-1))/2
  Initial : Constant  Value=0
  Integrator : Integrator  InitialCondition=-1.000
  Mul{1..18} (18 alike) : Product  Inputs=**  OutScaling=2^-10
  Output : Outport
  InputPass : Outport  Port=2
  State : Outport  Port=3
  wires:
  Add/1 -> 1/C/1
  1/C/1 -> Integrator/1
  Initial/1 -> Add/4
  1/R/1 -> Add/1
  Integrator/1 -> 1/R/1, F/1, State/1
  A1,1/1 -> Mul1/1
  Vyi-1,j-1/1 -> Mul1/2
  A1,2/1 -> Mul2/1
  Vyi-1,j/1 -> Mul2/2
  A1,3/1 -> Mul3/1
  Vyi-1,j+1/1 -> Mul3/2
  A2,1/1 -> Mul4/1
  Vyi,j-1/1 -> Mul4/2
  A2,2/1 -> Mul5/1
  A2,3/1 -> Mul6/1
  Vyi,j+1/1 -> Mul6/2
  A3,1/1 -> Mul7/1
  Vyi+1,j-1/1 -> Mul7/2
  A3,2/1 -> Mul8/1
  Vyi+1,j/1 -> Mul8/2
  A3,3/1 -> Mul9/1
  Vyi+1,j+1/1 -> Mul9/2
  F/1 -> Mul5/2, Output/1
  Mul3/1 -> Add1/1
  Mul6/1 -> Add1/2
  Mul9/1 -> Add1/3
  Mul2/1 -> Add1/4
  Mul5/1 -> Add1/5
  Mul8/1 -> Add1/6
  Mul1/1 -> Add1/7
  Mul4/1 -> Add1/8
  Mul7/1 -> Add1/9
  Add1/1 -> Add/2
  B1,1/1 -> Mul10/1
  Vui-1,j-1/1 -> Mul10/2
  B1,2/1 -> Mul11/1
  Vui-1,j/1 -> Mul11/2
  B1,3/1 -> Mul12/1
  Vui-1,j+1/1 -> Mul12/2
  B2,1/1 -> Mul13/1
  Vui,j-1/1 -> Mul13/2
  B2,2/1 -> Mul14/1
  B2,3/1 -> Mul15/1
  Vui,j+1/1 -> Mul15/2
  B3,1/1 -> Mul16/1
  Vui+1,j-1/1 -> Mul16/2
  B3,2/1 -> Mul17/1
  Vui+1,j/1 -> Mul17/2
  B3,3/1 -> Mul18/1
  Vui+1,j+1/1 -> Mul18/2
  Mul10/1 -> Add2/1
  Mul13/1 -> Add2/2
  Mul16/1 -> Add2/3
  Mul11/1 -> Add2/4
  Mul14/1 -> Add2/5
  Mul17/1 -> Add2/6
  Mul12/1 -> Add2/7
  Mul15/1 -> Add2/8
  Mul18/1 -> Add2/9
  Input/1 -> Mul14/2, InputPass/1
  Add2/1 -> Add/3

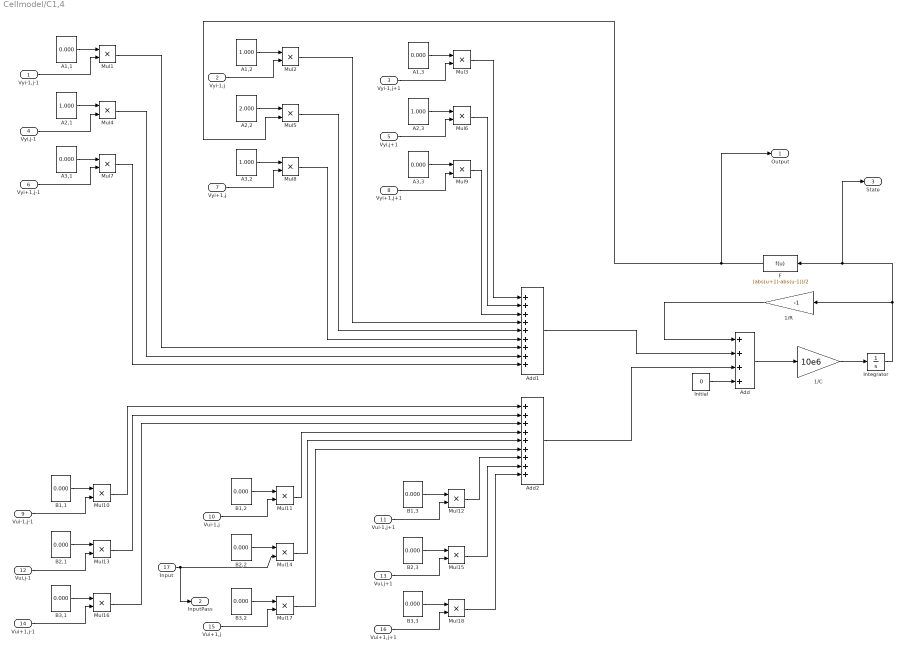
== system Cellmodel/C1,4 ==
  Vyi-1,j-1 : Inport
  Vyi-1,j : Inport  Port=2
  Vyi-1,j+1 : Inport  Port=3
  Vyi,j-1 : Inport  Port=4
  Vyi,j+1 : Inport  Port=5
  Vyi+1,j-1 : Inport  Port=6
  Vyi+1,j : Inport  Port=7
  Vyi+1,j+1 : Inport  Port=8
  Vui-1,j-1 : Inport  Port=9
  Vui-1,j : Inport  Port=10
  Vui-1,j+1 : Inport  Port=11
  Vui,j-1 : Inport  Port=12
  Vui,j+1 : Inport  Port=13
  Vui+1,j-1 : Inport  Port=14
  Vui+1,j : Inport  Port=15
  Vui+1,j+1 : Inport  Port=16
  Input : Inport  Port=17
  1/C : Gain  Gain=10e6
  1/R : Gain  Orientation=left  Gain=-1
  A1,1 : Constant  Value=0.000
  A1,2 : Constant  Value=1.000
  A1,3 : Constant  Value=0.000
  A2,1 : Constant  Value=1.000
  A2,2 : Constant  Value=2.000
  A2,3 : Constant  Value=1.000
  A3,1 : Constant  Value=0.000
  A3,2 : Constant  Value=1.000
  A3,3 : Constant  Value=0.000
  Add : Sum  Inputs=++++  OutScaling=2^-10
  Add1 : Sum  Inputs=+++++++++  OutScaling=2^-10
  Add2 : Sum  Inputs=+++++++++  OutScaling=2^-10
  B1,1 : Constant  Value=0.000
  B1,2 : Constant  Value=0.000
  B1,3 : Constant  Value=0.000
  B2,1 : Constant  Value=0.000
  B2,2 : Constant  Value=0.000
  B2,3 : Constant  Value=0.000
  B3,1 : Constant  Value=0.000
  B3,2 : Constant  Value=0.000
  B3,3 : Constant  Value=0.000
  F : Fcn  Orientation=left  Expr=(abs(u+1)-abs(u-1))/2
  Initial : Constant  Value=0
  Integrator : Integrator  InitialCondition=-0.600
  Mul{1..18} (18 alike) : Product  Inputs=**  OutScaling=2^-10
  Output : Outport
  InputPass : Outport  Port=2
  State : Outport  Port=3
  wires:
  Add2/1 -> Add/3
  Input/1 -> InputPass/1, Mul14/2
  Mul18/1 -> Add2/9
  Mul15/1 -> Add2/8
  Mul12/1 -> Add2/7
  Mul17/1 -> Add2/6
  Mul14/1 -> Add2/5
  Mul11/1 -> Add2/4
  Mul16/1 -> Add2/3
  Mul13/1 -> Add2/2
  Mul10/1 -> Add2/1
  Vui+1,j+1/1 -> Mul18/2
  B3,3/1 -> Mul18/1
  Vui+1,j/1 -> Mul17/2
  B3,2/1 -> Mul17/1
  Vui+1,j-1/1 -> Mul16/2
  B3,1/1 -> Mul16/1
  Vui,j+1/1 -> Mul15/2
  B2,3/1 -> Mul15/1
  B2,2/1 -> Mul14/1
  Vui,j-1/1 -> Mul13/2
  B2,1/1 -> Mul13/1
  Vui-1,j+1/1 -> Mul12/2
  B1,3/1 -> Mul12/1
  Vui-1,j/1 -> Mul11/2
  B1,2/1 -> Mul11/1
  Vui-1,j-1/1 -> Mul10/2
  B1,1/1 -> Mul10/1
  Add1/1 -> Add/2
  Mul7/1 -> Add1/9
  Mul4/1 -> Add1/8
  Mul1/1 -> Add1/7
  Mul8/1 -> Add1/6
  Mul5/1 -> Add1/5
  Mul2/1 -> Add1/4
  Mul9/1 -> Add1/3
  Mul6/1 -> Add1/2
  Mul3/1 -> Add1/1
  F/1 -> Mul5/2, Output/1
  Vyi+1,j+1/1 -> Mul9/2
  A3,3/1 -> Mul9/1
  Vyi+1,j/1 -> Mul8/2
  A3,2/1 -> Mul8/1
  Vyi+1,j-1/1 -> Mul7/2
  A3,1/1 -> Mul7/1
  Vyi,j+1/1 -> Mul6/2
  A2,3/1 -> Mul6/1
  A2,2/1 -> Mul5/1
  Vyi,j-1/1 -> Mul4/2
  A2,1/1 -> Mul4/1
  Vyi-1,j+1/1 -> Mul3/2
  A1,3/1 -> Mul3/1
  Vyi-1,j/1 -> Mul2/2
  A1,2/1 -> Mul2/1
  Vyi-1,j-1/1 -> Mul1/2
  A1,1/1 -> Mul1/1
  Integrator/1 -> 1/R/1, F/1, State/1
  1/R/1 -> Add/1
  Initial/1 -> Add/4
  1/C/1 -> Integrator/1
  Add/1 -> 1/C/1

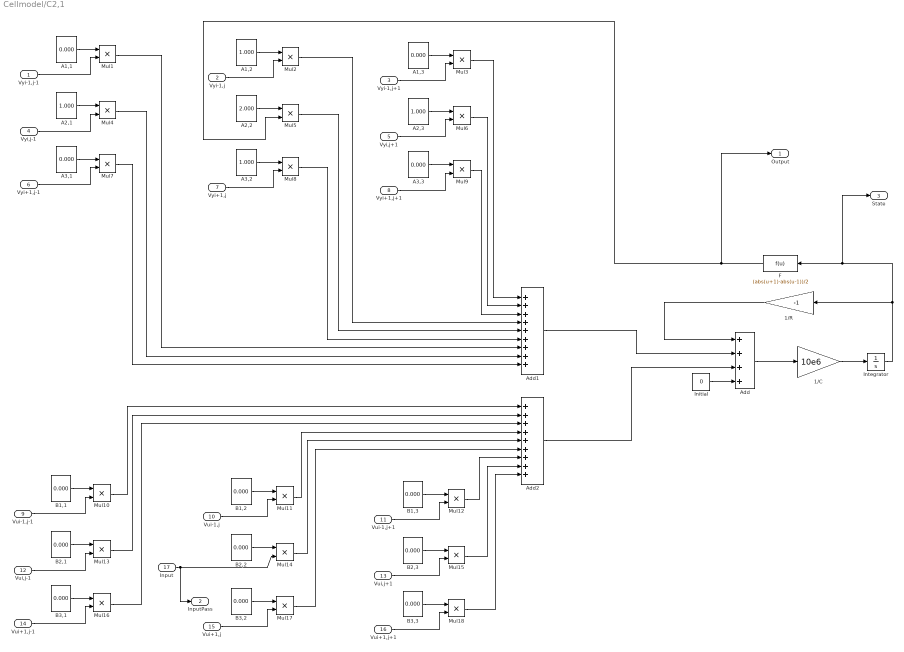
== system Cellmodel/C2,1 ==
  Vyi-1,j-1 : Inport
  Vyi-1,j : Inport  Port=2
  Vyi-1,j+1 : Inport  Port=3
  Vyi,j-1 : Inport  Port=4
  Vyi,j+1 : Inport  Port=5
  Vyi+1,j-1 : Inport  Port=6
  Vyi+1,j : Inport  Port=7
  Vyi+1,j+1 : Inport  Port=8
  Vui-1,j-1 : Inport  Port=9
  Vui-1,j : Inport  Port=10
  Vui-1,j+1 : Inport  Port=11
  Vui,j-1 : Inport  Port=12
  Vui,j+1 : Inport  Port=13
  Vui+1,j-1 : Inport  Port=14
  Vui+1,j : Inport  Port=15
  Vui+1,j+1 : Inport  Port=16
  Input : Inport  Port=17
  1/C : Gain  Gain=10e6
  1/R : Gain  Orientation=left  Gain=-1
  A1,1 : Constant  Value=0.000
  A1,2 : Constant  Value=1.000
  A1,3 : Constant  Value=0.000
  A2,1 : Constant  Value=1.000
  A2,2 : Constant  Value=2.000
  A2,3 : Constant  Value=1.000
  A3,1 : Constant  Value=0.000
  A3,2 : Constant  Value=1.000
  A3,3 : Constant  Value=0.000
  Add : Sum  Inputs=++++  OutScaling=2^-10
  Add1 : Sum  Inputs=+++++++++  OutScaling=2^-10
  Add2 : Sum  Inputs=+++++++++  OutScaling=2^-10
  B1,1 : Constant  Value=0.000
  B1,2 : Constant  Value=0.000
  B1,3 : Constant  Value=0.000
  B2,1 : Constant  Value=0.000
  B2,2 : Constant  Value=0.000
  B2,3 : Constant  Value=0.000
  B3,1 : Constant  Value=0.000
  B3,2 : Constant  Value=0.000
  B3,3 : Constant  Value=0.000
  F : Fcn  Orientation=left  Expr=(abs(u+1)-abs(u-1))/2
  Initial : Constant  Value=0
  Integrator : Integrator  InitialCondition=1.000
  Mul{1..18} (18 alike) : Product  Inputs=**  OutScaling=2^-10
  Output : Outport
  InputPass : Outport  Port=2
  State : Outport  Port=3
  wires:
  Add2/1 -> Add/3
  Input/1 -> InputPass/1, Mul14/2
  Mul18/1 -> Add2/9
  Mul15/1 -> Add2/8
  Mul12/1 -> Add2/7
  Mul17/1 -> Add2/6
  Mul14/1 -> Add2/5
  Mul11/1 -> Add2/4
  Mul16/1 -> Add2/3
  Mul13/1 -> Add2/2
  Mul10/1 -> Add2/1
  Vui+1,j+1/1 -> Mul18/2
  B3,3/1 -> Mul18/1
  Vui+1,j/1 -> Mul17/2
  B3,2/1 -> Mul17/1
  Vui+1,j-1/1 -> Mul16/2
  B3,1/1 -> Mul16/1
  Vui,j+1/1 -> Mul15/2
  B2,3/1 -> Mul15/1
  B2,2/1 -> Mul14/1
  Vui,j-1/1 -> Mul13/2
  B2,1/1 -> Mul13/1
  Vui-1,j+1/1 -> Mul12/2
  B1,3/1 -> Mul12/1
  Vui-1,j/1 -> Mul11/2
  B1,2/1 -> Mul11/1
  Vui-1,j-1/1 -> Mul10/2
  B1,1/1 -> Mul10/1
  Add1/1 -> Add/2
  Mul7/1 -> Add1/9
  Mul4/1 -> Add1/8
  Mul1/1 -> Add1/7
  Mul8/1 -> Add1/6
  Mul5/1 -> Add1/5
  Mul2/1 -> Add1/4
  Mul9/1 -> Add1/3
  Mul6/1 -> Add1/2
  Mul3/1 -> Add1/1
  F/1 -> Mul5/2, Output/1
  Vyi+1,j+1/1 -> Mul9/2
  A3,3/1 -> Mul9/1
  Vyi+1,j/1 -> Mul8/2
  A3,2/1 -> Mul8/1
  Vyi+1,j-1/1 -> Mul7/2
  A3,1/1 -> Mul7/1
  Vyi,j+1/1 -> Mul6/2
  A2,3/1 -> Mul6/1
  A2,2/1 -> Mul5/1
  Vyi,j-1/1 -> Mul4/2
  A2,1/1 -> Mul4/1
  Vyi-1,j+1/1 -> Mul3/2
  A1,3/1 -> Mul3/1
  Vyi-1,j/1 -> Mul2/2
  A1,2/1 -> Mul2/1
  Vyi-1,j-1/1 -> Mul1/2
  A1,1/1 -> Mul1/1
  Integrator/1 -> 1/R/1, F/1, State/1
  1/R/1 -> Add/1
  Initial/1 -> Add/4
  1/C/1 -> Integrator/1
  Add/1 -> 1/C/1

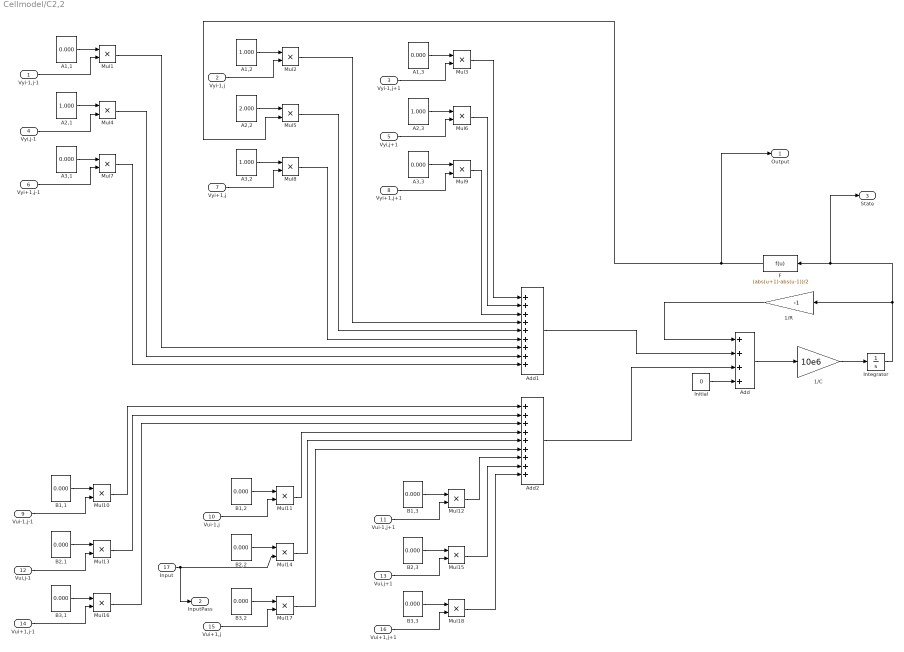
== system Cellmodel/C2,2 ==
  Vyi-1,j-1 : Inport
  Vyi-1,j : Inport  Port=2
  Vyi-1,j+1 : Inport  Port=3
  Vyi,j-1 : Inport  Port=4
  Vyi,j+1 : Inport  Port=5
  Vyi+1,j-1 : Inport  Port=6
  Vyi+1,j : Inport  Port=7
  Vyi+1,j+1 : Inport  Port=8
  Vui-1,j-1 : Inport  Port=9
  Vui-1,j : Inport  Port=10
  Vui-1,j+1 : Inport  Port=11
  Vui,j-1 : Inport  Port=12
  Vui,j+1 : Inport  Port=13
  Vui+1,j-1 : Inport  Port=14
  Vui+1,j : Inport  Port=15
  Vui+1,j+1 : Inport  Port=16
  Input : Inport  Port=17
  1/C : Gain  Gain=10e6
  1/R : Gain  Orientation=left  Gain=-1
  A1,1 : Constant  Value=0.000
  A1,2 : Constant  Value=1.000
  A1,3 : Constant  Value=0.000
  A2,1 : Constant  Value=1.000
  A2,2 : Constant  Value=2.000
  A2,3 : Constant  Value=1.000
  A3,1 : Constant  Value=0.000
  A3,2 : Constant  Value=1.000
  A3,3 : Constant  Value=0.000
  Add : Sum  Inputs=++++  OutScaling=2^-10
  Add1 : Sum  Inputs=+++++++++  OutScaling=2^-10
  Add2 : Sum  Inputs=+++++++++  OutScaling=2^-10
  B1,1 : Constant  Value=0.000
  B1,2 : Constant  Value=0.000
  B1,3 : Constant  Value=0.000
  B2,1 : Constant  Value=0.000
  B2,2 : Constant  Value=0.000
  B2,3 : Constant  Value=0.000
  B3,1 : Constant  Value=0.000
  B3,2 : Constant  Value=0.000
  B3,3 : Constant  Value=0.000
  F : Fcn  Orientation=left  Expr=(abs(u+1)-abs(u-1))/2
  Initial : Constant  Value=0
  Integrator : Integrator  InitialCondition=1.000
  Mul{1..18} (18 alike) : Product  Inputs=**  OutScaling=2^-10
  Output : Outport
  InputPass : Outport  Port=2
  State : Outport  Port=3
  wires:
  Add/1 -> 1/C/1
  1/C/1 -> Integrator/1
  Initial/1 -> Add/4
  1/R/1 -> Add/1
  Integrator/1 -> 1/R/1, F/1, State/1
  A1,1/1 -> Mul1/1
  Vyi-1,j-1/1 -> Mul1/2
  A1,2/1 -> Mul2/1
  Vyi-1,j/1 -> Mul2/2
  A1,3/1 -> Mul3/1
  Vyi-1,j+1/1 -> Mul3/2
  A2,1/1 -> Mul4/1
  Vyi,j-1/1 -> Mul4/2
  A2,2/1 -> Mul5/1
  A2,3/1 -> Mul6/1
  Vyi,j+1/1 -> Mul6/2
  A3,1/1 -> Mul7/1
  Vyi+1,j-1/1 -> Mul7/2
  A3,2/1 -> Mul8/1
  Vyi+1,j/1 -> Mul8/2
  A3,3/1 -> Mul9/1
  Vyi+1,j+1/1 -> Mul9/2
  F/1 -> Mul5/2, Output/1
  Mul3/1 -> Add1/1
  Mul6/1 -> Add1/2
  Mul9/1 -> Add1/3
  Mul2/1 -> Add1/4
  Mul5/1 -> Add1/5
  Mul8/1 -> Add1/6
  Mul1/1 -> Add1/7
  Mul4/1 -> Add1/8
  Mul7/1 -> Add1/9
  Add1/1 -> Add/2
  B1,1/1 -> Mul10/1
  Vui-1,j-1/1 -> Mul10/2
  B1,2/1 -> Mul11/1
  Vui-1,j/1 -> Mul11/2
  B1,3/1 -> Mul12/1
  Vui-1,j+1/1 -> Mul12/2
  B2,1/1 -> Mul13/1
  Vui,j-1/1 -> Mul13/2
  B2,2/1 -> Mul14/1
  B2,3/1 -> Mul15/1
  Vui,j+1/1 -> Mul15/2
  B3,1/1 -> Mul16/1
  Vui+1,j-1/1 -> Mul16/2
  B3,2/1 -> Mul17/1
  Vui+1,j/1 -> Mul17/2
  B3,3/1 -> Mul18/1
  Vui+1,j+1/1 -> Mul18/2
  Mul10/1 -> Add2/1
  Mul13/1 -> Add2/2
  Mul16/1 -> Add2/3
  Mul11/1 -> Add2/4
  Mul14/1 -> Add2/5
  Mul17/1 -> Add2/6
  Mul12/1 -> Add2/7
  Mul15/1 -> Add2/8
  Mul18/1 -> Add2/9
  Input/1 -> Mul14/2, InputPass/1
  Add2/1 -> Add/3

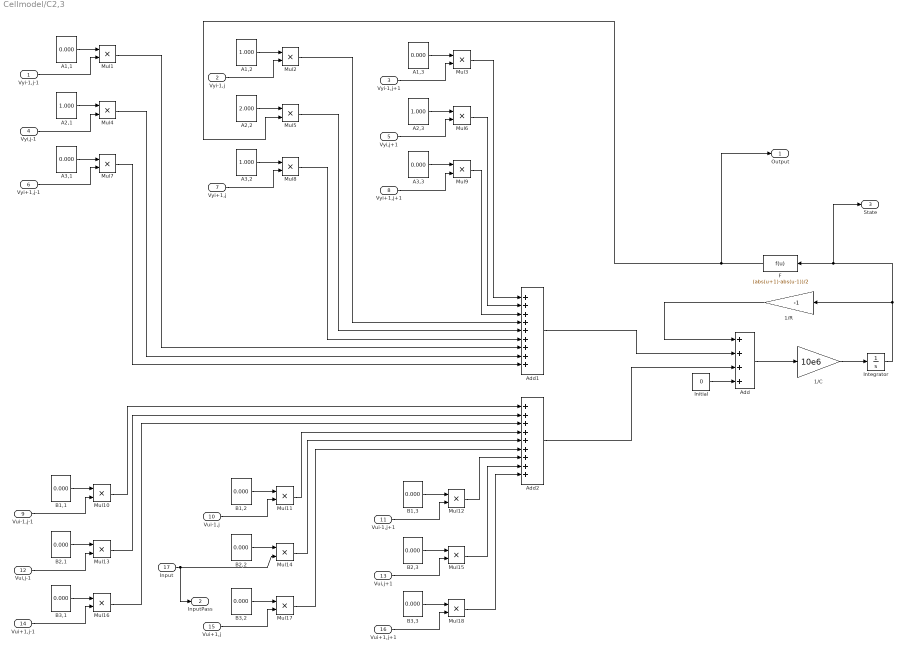
== system Cellmodel/C2,3 ==
  Vyi-1,j-1 : Inport
  Vyi-1,j : Inport  Port=2
  Vyi-1,j+1 : Inport  Port=3
  Vyi,j-1 : Inport  Port=4
  Vyi,j+1 : Inport  Port=5
  Vyi+1,j-1 : Inport  Port=6
  Vyi+1,j : Inport  Port=7
  Vyi+1,j+1 : Inport  Port=8
  Vui-1,j-1 : Inport  Port=9
  Vui-1,j : Inport  Port=10
  Vui-1,j+1 : Inport  Port=11
  Vui,j-1 : Inport  Port=12
  Vui,j+1 : Inport  Port=13
  Vui+1,j-1 : Inport  Port=14
  Vui+1,j : Inport  Port=15
  Vui+1,j+1 : Inport  Port=16
  Input : Inport  Port=17
  1/C : Gain  Gain=10e6
  1/R : Gain  Orientation=left  Gain=-1
  A1,1 : Constant  Value=0.000
  A1,2 : Constant  Value=1.000
  A1,3 : Constant  Value=0.000
  A2,1 : Constant  Value=1.000
  A2,2 : Constant  Value=2.000
  A2,3 : Constant  Value=1.000
  A3,1 : Constant  Value=0.000
  A3,2 : Constant  Value=1.000
  A3,3 : Constant  Value=0.000
  Add : Sum  Inputs=++++  OutScaling=2^-10
  Add1 : Sum  Inputs=+++++++++  OutScaling=2^-10
  Add2 : Sum  Inputs=+++++++++  OutScaling=2^-10
  B1,1 : Constant  Value=0.000
  B1,2 : Constant  Value=0.000
  B1,3 : Constant  Value=0.000
  B2,1 : Constant  Value=0.000
  B2,2 : Constant  Value=0.000
  B2,3 : Constant  Value=0.000
  B3,1 : Constant  Value=0.000
  B3,2 : Constant  Value=0.000
  B3,3 : Constant  Value=0.000
  F : Fcn  Orientation=left  Expr=(abs(u+1)-abs(u-1))/2
  Initial : Constant  Value=0
  Integrator : Integrator  InitialCondition=1.000
  Mul{1..18} (18 alike) : Product  Inputs=**  OutScaling=2^-10
  Output : Outport
  InputPass : Outport  Port=2
  State : Outport  Port=3
  wires:
  Add2/1 -> Add/3
  Input/1 -> InputPass/1, Mul14/2
  Mul18/1 -> Add2/9
  Mul15/1 -> Add2/8
  Mul12/1 -> Add2/7
  Mul17/1 -> Add2/6
  Mul14/1 -> Add2/5
  Mul11/1 -> Add2/4
  Mul16/1 -> Add2/3
  Mul13/1 -> Add2/2
  Mul10/1 -> Add2/1
  Vui+1,j+1/1 -> Mul18/2
  B3,3/1 -> Mul18/1
  Vui+1,j/1 -> Mul17/2
  B3,2/1 -> Mul17/1
  Vui+1,j-1/1 -> Mul16/2
  B3,1/1 -> Mul16/1
  Vui,j+1/1 -> Mul15/2
  B2,3/1 -> Mul15/1
  B2,2/1 -> Mul14/1
  Vui,j-1/1 -> Mul13/2
  B2,1/1 -> Mul13/1
  Vui-1,j+1/1 -> Mul12/2
  B1,3/1 -> Mul12/1
  Vui-1,j/1 -> Mul11/2
  B1,2/1 -> Mul11/1
  Vui-1,j-1/1 -> Mul10/2
  B1,1/1 -> Mul10/1
  Add1/1 -> Add/2
  Mul7/1 -> Add1/9
  Mul4/1 -> Add1/8
  Mul1/1 -> Add1/7
  Mul8/1 -> Add1/6
  Mul5/1 -> Add1/5
  Mul2/1 -> Add1/4
  Mul9/1 -> Add1/3
  Mul6/1 -> Add1/2
  Mul3/1 -> Add1/1
  F/1 -> Mul5/2, Output/1
  Vyi+1,j+1/1 -> Mul9/2
  A3,3/1 -> Mul9/1
  Vyi+1,j/1 -> Mul8/2
  A3,2/1 -> Mul8/1
  Vyi+1,j-1/1 -> Mul7/2
  A3,1/1 -> Mul7/1
  Vyi,j+1/1 -> Mul6/2
  A2,3/1 -> Mul6/1
  A2,2/1 -> Mul5/1
  Vyi,j-1/1 -> Mul4/2
  A2,1/1 -> Mul4/1
  Vyi-1,j+1/1 -> Mul3/2
  A1,3/1 -> Mul3/1
  Vyi-1,j/1 -> Mul2/2
  A1,2/1 -> Mul2/1
  Vyi-1,j-1/1 -> Mul1/2
  A1,1/1 -> Mul1/1
  Integrator/1 -> 1/R/1, F/1, State/1
  1/R/1 -> Add/1
  Initial/1 -> Add/4
  1/C/1 -> Integrator/1
  Add/1 -> 1/C/1

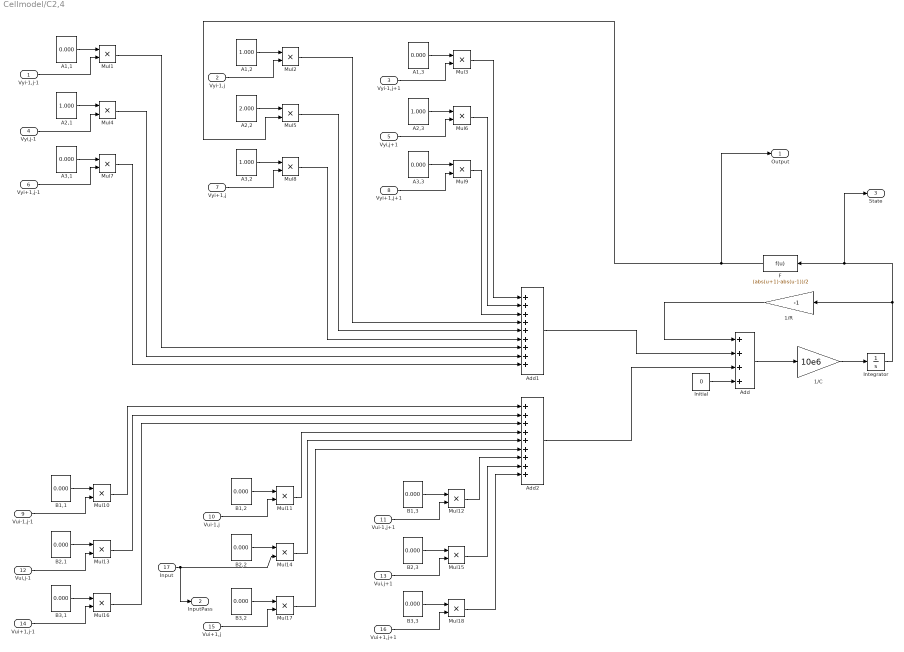
== system Cellmodel/C2,4 ==
  Vyi-1,j-1 : Inport
  Vyi-1,j : Inport  Port=2
  Vyi-1,j+1 : Inport  Port=3
  Vyi,j-1 : Inport  Port=4
  Vyi,j+1 : Inport  Port=5
  Vyi+1,j-1 : Inport  Port=6
  Vyi+1,j : Inport  Port=7
  Vyi+1,j+1 : Inport  Port=8
  Vui-1,j-1 : Inport  Port=9
  Vui-1,j : Inport  Port=10
  Vui-1,j+1 : Inport  Port=11
  Vui,j-1 : Inport  Port=12
  Vui,j+1 : Inport  Port=13
  Vui+1,j-1 : Inport  Port=14
  Vui+1,j : Inport  Port=15
  Vui+1,j+1 : Inport  Port=16
  Input : Inport  Port=17
  1/C : Gain  Gain=10e6
  1/R : Gain  Orientation=left  Gain=-1
  A1,1 : Constant  Value=0.000
  A1,2 : Constant  Value=1.000
  A1,3 : Constant  Value=0.000
  A2,1 : Constant  Value=1.000
  A2,2 : Constant  Value=2.000
  A2,3 : Constant  Value=1.000
  A3,1 : Constant  Value=0.000
  A3,2 : Constant  Value=1.000
  A3,3 : Constant  Value=0.000
  Add : Sum  Inputs=++++  OutScaling=2^-10
  Add1 : Sum  Inputs=+++++++++  OutScaling=2^-10
  Add2 : Sum  Inputs=+++++++++  OutScaling=2^-10
  B1,1 : Constant  Value=0.000
  B1,2 : Constant  Value=0.000
  B1,3 : Constant  Value=0.000
  B2,1 : Constant  Value=0.000
  B2,2 : Constant  Value=0.000
  B2,3 : Constant  Value=0.000
  B3,1 : Constant  Value=0.000
  B3,2 : Constant  Value=0.000
  B3,3 : Constant  Value=0.000
  F : Fcn  Orientation=left  Expr=(abs(u+1)-abs(u-1))/2
  Initial : Constant  Value=0
  Integrator : Integrator  InitialCondition=-1.000
  Mul{1..18} (18 alike) : Product  Inputs=**  OutScaling=2^-10
  Output : Outport
  InputPass : Outport  Port=2
  State : Outport  Port=3
  wires:
  Add/1 -> 1/C/1
  1/C/1 -> Integrator/1
  Initial/1 -> Add/4
  1/R/1 -> Add/1
  Integrator/1 -> 1/R/1, F/1, State/1
  A1,1/1 -> Mul1/1
  Vyi-1,j-1/1 -> Mul1/2
  A1,2/1 -> Mul2/1
  Vyi-1,j/1 -> Mul2/2
  A1,3/1 -> Mul3/1
  Vyi-1,j+1/1 -> Mul3/2
  A2,1/1 -> Mul4/1
  Vyi,j-1/1 -> Mul4/2
  A2,2/1 -> Mul5/1
  A2,3/1 -> Mul6/1
  Vyi,j+1/1 -> Mul6/2
  A3,1/1 -> Mul7/1
  Vyi+1,j-1/1 -> Mul7/2
  A3,2/1 -> Mul8/1
  Vyi+1,j/1 -> Mul8/2
  A3,3/1 -> Mul9/1
  Vyi+1,j+1/1 -> Mul9/2
  F/1 -> Mul5/2, Output/1
  Mul3/1 -> Add1/1
  Mul6/1 -> Add1/2
  Mul9/1 -> Add1/3
  Mul2/1 -> Add1/4
  Mul5/1 -> Add1/5
  Mul8/1 -> Add1/6
  Mul1/1 -> Add1/7
  Mul4/1 -> Add1/8
  Mul7/1 -> Add1/9
  Add1/1 -> Add/2
  B1,1/1 -> Mul10/1
  Vui-1,j-1/1 -> Mul10/2
  B1,2/1 -> Mul11/1
  Vui-1,j/1 -> Mul11/2
  B1,3/1 -> Mul12/1
  Vui-1,j+1/1 -> Mul12/2
  B2,1/1 -> Mul13/1
  Vui,j-1/1 -> Mul13/2
  B2,2/1 -> Mul14/1
  B2,3/1 -> Mul15/1
  Vui,j+1/1 -> Mul15/2
  B3,1/1 -> Mul16/1
  Vui+1,j-1/1 -> Mul16/2
  B3,2/1 -> Mul17/1
  Vui+1,j/1 -> Mul17/2
  B3,3/1 -> Mul18/1
  Vui+1,j+1/1 -> Mul18/2
  Mul10/1 -> Add2/1
  Mul13/1 -> Add2/2
  Mul16/1 -> Add2/3
  Mul11/1 -> Add2/4
  Mul14/1 -> Add2/5
  Mul17/1 -> Add2/6
  Mul12/1 -> Add2/7
  Mul15/1 -> Add2/8
  Mul18/1 -> Add2/9
  Input/1 -> Mul14/2, InputPass/1
  Add2/1 -> Add/3

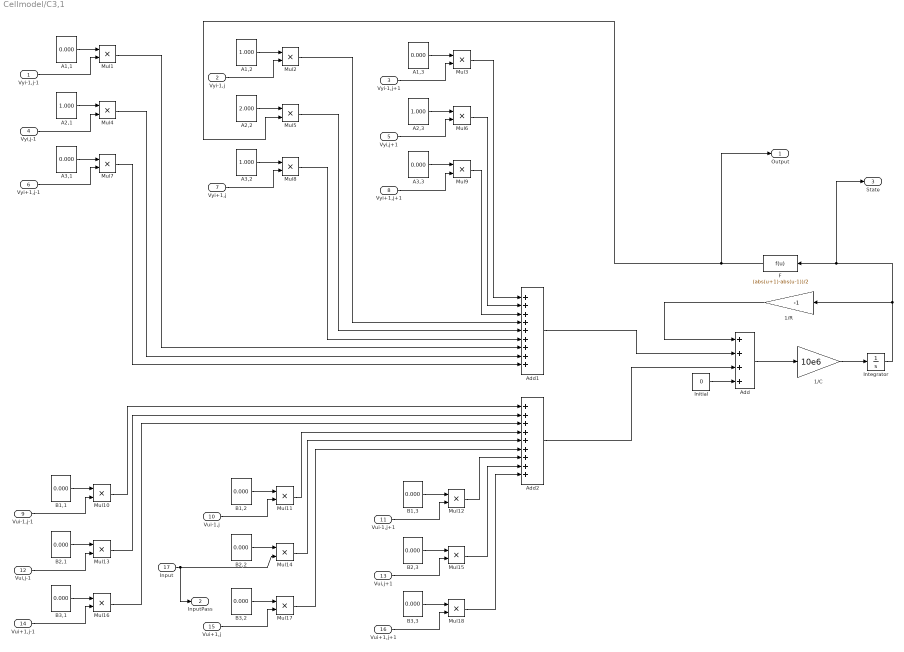
== system Cellmodel/C3,1 ==
  Vyi-1,j-1 : Inport
  Vyi-1,j : Inport  Port=2
  Vyi-1,j+1 : Inport  Port=3
  Vyi,j-1 : Inport  Port=4
  Vyi,j+1 : Inport  Port=5
  Vyi+1,j-1 : Inport  Port=6
  Vyi+1,j : Inport  Port=7
  Vyi+1,j+1 : Inport  Port=8
  Vui-1,j-1 : Inport  Port=9
  Vui-1,j : Inport  Port=10
  Vui-1,j+1 : Inport  Port=11
  Vui,j-1 : Inport  Port=12
  Vui,j+1 : Inport  Port=13
  Vui+1,j-1 : Inport  Port=14
  Vui+1,j : Inport  Port=15
  Vui+1,j+1 : Inport  Port=16
  Input : Inport  Port=17
  1/C : Gain  Gain=10e6
  1/R : Gain  Orientation=left  Gain=-1
  A1,1 : Constant  Value=0.000
  A1,2 : Constant  Value=1.000
  A1,3 : Constant  Value=0.000
  A2,1 : Constant  Value=1.000
  A2,2 : Constant  Value=2.000
  A2,3 : Constant  Value=1.000
  A3,1 : Constant  Value=0.000
  A3,2 : Constant  Value=1.000
  A3,3 : Constant  Value=0.000
  Add : Sum  Inputs=++++  OutScaling=2^-10
  Add1 : Sum  Inputs=+++++++++  OutScaling=2^-10
  Add2 : Sum  Inputs=+++++++++  OutScaling=2^-10
  B1,1 : Constant  Value=0.000
  B1,2 : Constant  Value=0.000
  B1,3 : Constant  Value=0.000
  B2,1 : Constant  Value=0.000
  B2,2 : Constant  Value=0.000
  B2,3 : Constant  Value=0.000
  B3,1 : Constant  Value=0.000
  B3,2 : Constant  Value=0.000
  B3,3 : Constant  Value=0.000
  F : Fcn  Orientation=left  Expr=(abs(u+1)-abs(u-1))/2
  Initial : Constant  Value=0
  Integrator : Integrator  InitialCondition=-1.000
  Mul{1..18} (18 alike) : Product  Inputs=**  OutScaling=2^-10
  Output : Outport
  InputPass : Outport  Port=2
  State : Outport  Port=3
  wires:
  Add/1 -> 1/C/1
  1/C/1 -> Integrator/1
  Initial/1 -> Add/4
  1/R/1 -> Add/1
  Integrator/1 -> 1/R/1, F/1, State/1
  A1,1/1 -> Mul1/1
  Vyi-1,j-1/1 -> Mul1/2
  A1,2/1 -> Mul2/1
  Vyi-1,j/1 -> Mul2/2
  A1,3/1 -> Mul3/1
  Vyi-1,j+1/1 -> Mul3/2
  A2,1/1 -> Mul4/1
  Vyi,j-1/1 -> Mul4/2
  A2,2/1 -> Mul5/1
  A2,3/1 -> Mul6/1
  Vyi,j+1/1 -> Mul6/2
  A3,1/1 -> Mul7/1
  Vyi+1,j-1/1 -> Mul7/2
  A3,2/1 -> Mul8/1
  Vyi+1,j/1 -> Mul8/2
  A3,3/1 -> Mul9/1
  Vyi+1,j+1/1 -> Mul9/2
  F/1 -> Mul5/2, Output/1
  Mul3/1 -> Add1/1
  Mul6/1 -> Add1/2
  Mul9/1 -> Add1/3
  Mul2/1 -> Add1/4
  Mul5/1 -> Add1/5
  Mul8/1 -> Add1/6
  Mul1/1 -> Add1/7
  Mul4/1 -> Add1/8
  Mul7/1 -> Add1/9
  Add1/1 -> Add/2
  B1,1/1 -> Mul10/1
  Vui-1,j-1/1 -> Mul10/2
  B1,2/1 -> Mul11/1
  Vui-1,j/1 -> Mul11/2
  B1,3/1 -> Mul12/1
  Vui-1,j+1/1 -> Mul12/2
  B2,1/1 -> Mul13/1
  Vui,j-1/1 -> Mul13/2
  B2,2/1 -> Mul14/1
  B2,3/1 -> Mul15/1
  Vui,j+1/1 -> Mul15/2
  B3,1/1 -> Mul16/1
  Vui+1,j-1/1 -> Mul16/2
  B3,2/1 -> Mul17/1
  Vui+1,j/1 -> Mul17/2
  B3,3/1 -> Mul18/1
  Vui+1,j+1/1 -> Mul18/2
  Mul10/1 -> Add2/1
  Mul13/1 -> Add2/2
  Mul16/1 -> Add2/3
  Mul11/1 -> Add2/4
  Mul14/1 -> Add2/5
  Mul17/1 -> Add2/6
  Mul12/1 -> Add2/7
  Mul15/1 -> Add2/8
  Mul18/1 -> Add2/9
  Input/1 -> Mul14/2, InputPass/1
  Add2/1 -> Add/3
